simulink model "Simulink_Deliverable"  (R2020a)
settings: Solver=FixedStepAuto  StartTime=0.0  StopTime=10.0  FixedStep=1e-3  RelTol=1e-3  EnableMultiTasking=on
undefined symbols (not defined in the file or in its folder): D0, D1, D10, D11, D12, D13, D2, D3, D4, D5, D6, D7, D8, D9, PTA0, PTA1, PTA2, PTB23, PTB9, PTC16, PTC17, PTC2, PTC3, PTC4, PTD0, PTD1, PTD2, PTD3
libraries: frdmk64flib x17
settings Model: ExtModeTrigDuration=5  Creator=shivr  LastModifiedBy=shivr
settings OptimizationCC: EnhancedBackFolding=on  PassReuseOutputArgsAs=Individual arguments  ZeroExternalMemoryAtStartup=off  ZeroInternalMemoryAtStartup=off  MaxStackSize=64  OptimizeBlockOrder=speed  DifferentSizesBufferReuse=on  OptimizationCustomize=off  EfficientTunableParamExpr=on
settings DebuggingCC: ParameterTunabilityLossMsg=error
settings HardwareCC: ProdBitPerPointer=32  ProdBitPerSizeT=32  ProdBitPerPtrDiffT=32  ProdLargestAtomicInteger=Long  ProdLargestAtomicFloat=Double  ProdWordSize=32  ProdHWDeviceType=ARM Compatible->ARM Cortex
settings SFSimCC: MATLABDynamicMemAlloc=off
settings RTWCC: SystemTargetFile=ert.tlc  HardwareBoard=NXP FRDM-K64F  TemplateMakefile=ert_default_tmf  Toolchain=GNU Tools for ARM Embedded Processors
settings CodeAppCC: ForceParamTrailComments=on  IgnoreCustomStorageClasses=off  OperatorAnnotations=on  SimulinkDataObjDesc=on  SFDataObjDesc=on  InsertBlockDesc=on

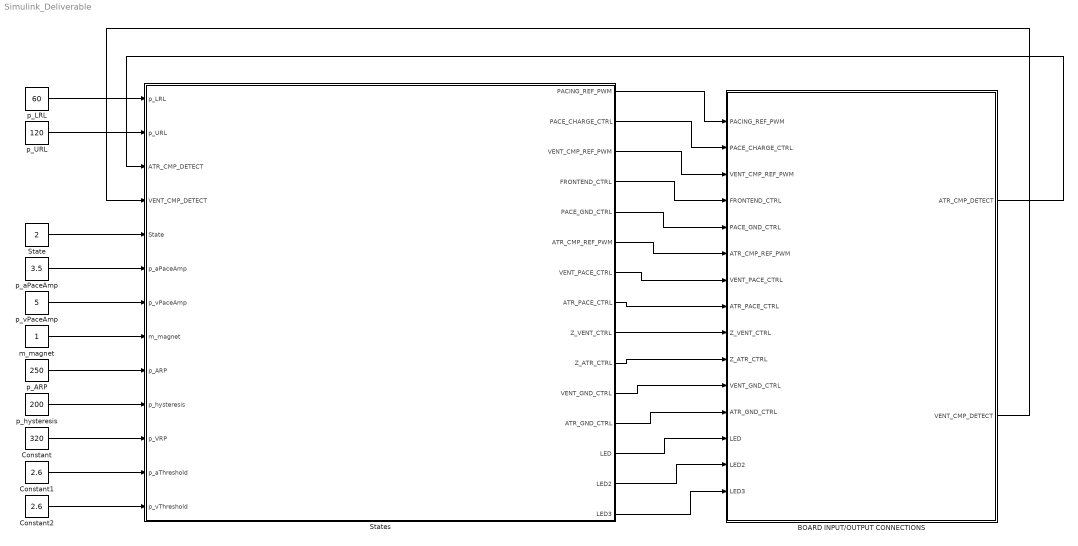
== system Simulink_Deliverable ==
  BOARD INPUT/OUTPUT CONNECTIONS : Subsystem
  Constant : Constant  Value=320
  Constant1 : Constant  Value=2.6
  Constant2 : Constant  Value=2.6
  State : Constant  Value=2
  States : Subsystem
  m_magnet : Constant
  p_ARP : Constant  Value=250
  p_LRL : Constant  Value=60
  p_URL : Constant  Value=120
  p_aPaceAmp : Constant  Value=3.5
  p_hysteresis : Constant  Value=200
  p_vPaceAmp : Constant  Value=5
  wires:
  p_LRL/1 -> States/1(p_LRL)
  States/12(ATR_GND_CTRL) -> BOARD INPUT/OUTPUT CONNECTIONS/12(ATR_GND_CTRL)
  States/5(PACE_GND_CTRL) -> BOARD INPUT/OUTPUT CONNECTIONS/5(PACE_GND_CTRL)
  States/11(VENT_GND_CTRL) -> BOARD INPUT/OUTPUT CONNECTIONS/11(VENT_GND_CTRL)
  States/7(VENT_PACE_CTRL) -> BOARD INPUT/OUTPUT CONNECTIONS/7(VENT_PACE_CTRL)
  States/8(ATR_PACE_CTRL) -> BOARD INPUT/OUTPUT CONNECTIONS/8(ATR_PACE_CTRL)
  States/9(Z_VENT_CTRL) -> BOARD INPUT/OUTPUT CONNECTIONS/9(Z_VENT_CTRL)
  States/10(Z_ATR_CTRL) -> BOARD INPUT/OUTPUT CONNECTIONS/10(Z_ATR_CTRL)
  States/4(FRONTEND_CTRL) -> BOARD INPUT/OUTPUT CONNECTIONS/4(FRONTEND_CTRL)
  States/2(PACE_CHARGE_CTRL) -> BOARD INPUT/OUTPUT CONNECTIONS/2(PACE_CHARGE_CTRL)
  States/1(PACING_REF_PWM) -> BOARD INPUT/OUTPUT CONNECTIONS/1(PACING_REF_PWM)
  States/13(LED) -> BOARD INPUT/OUTPUT CONNECTIONS/13(LED)
  p_URL/1 -> States/2(p_URL)
  BOARD INPUT/OUTPUT CONNECTIONS/1(ATR_CMP_DETECT) -> States/3(ATR_CMP_DETECT)
  BOARD INPUT/OUTPUT CONNECTIONS/2(VENT_CMP_DETECT) -> States/4(VENT_CMP_DETECT)
  p_aPaceAmp/1 -> States/6(p_aPaceAmp)
  m_magnet/1 -> States/8(m_magnet)
  States/14(LED2) -> BOARD INPUT/OUTPUT CONNECTIONS/14(LED2)
  p_vPaceAmp/1 -> States/7(p_vPaceAmp)
  States/6(ATR_CMP_REF_PWM) -> BOARD INPUT/OUTPUT CONNECTIONS/6(ATR_CMP_REF_PWM)
  p_ARP/1 -> States/9(p_ARP)
  p_hysteresis/1 -> States/10(p_hysteresis)
  States/15(LED3) -> BOARD INPUT/OUTPUT CONNECTIONS/15(LED3)
  States/3(VENT_CMP_REF_PWM) -> BOARD INPUT/OUTPUT CONNECTIONS/3(VENT_CMP_REF_PWM)
  Constant/1 -> States/11(p_VRP)
  Constant1/1 -> States/12(p_aThreshold)
  Constant2/1 -> States/13(p_vThreshold)
  State/1 -> States/5(State)

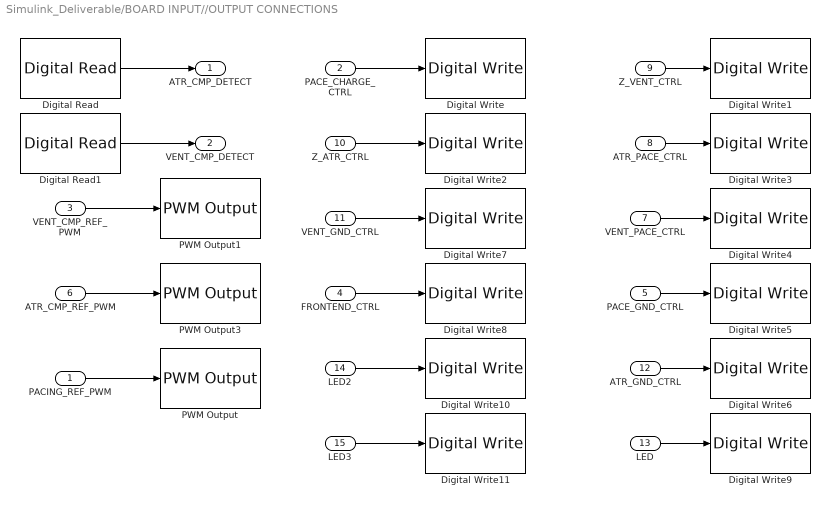
== system Simulink_Deliverable/BOARD INPUT//OUTPUT CONNECTIONS ==
  PACING_REF_PWM : Inport
  PACE_CHARGE_CTRL : Inport  Port=2
  VENT_CMP_REF_PWM : Inport  Port=3
  FRONTEND_CTRL : Inport  Port=4
  PACE_GND_CTRL : Inport  Port=5
  ATR_CMP_REF_PWM : Inport  Port=6
  VENT_PACE_CTRL : Inport  Port=7
  ATR_PACE_CTRL : Inport  Port=8
  Z_VENT_CTRL : Inport  Port=9
  Z_ATR_CTRL : Inport  Port=10
  VENT_GND_CTRL : Inport  Port=11
  ATR_GND_CTRL : Inport  Port=12
  LED : Inport  Port=13
  LED2 : Inport  Port=14
  LED3 : Inport  Port=15
  Digital Read : frdmk64flib/Digital Read  Whichpin=PTC16 (D0)  SampleTime=-1
  Digital Read1 : frdmk64flib/Digital Read  Whichpin=PTC17 (D1)  SampleTime=-1
  Digital Write : frdmk64flib/Digital Write  Whichpin=PTB9 (D2)
  Digital Write1 : frdmk64flib/Digital Write  Whichpin=PTC3 (D7)
  Digital Write10 : frdmk64flib/Digital Write  Whichpin=BLUE_LED
  Digital Write11 : frdmk64flib/Digital Write  Whichpin=GREEN_LED
  Digital Write2 : frdmk64flib/Digital Write  Whichpin=PTB23 (D4)
  Digital Write3 : frdmk64flib/Digital Write  Whichpin=PTA0 (D8)
  Digital Write4 : frdmk64flib/Digital Write  Whichpin=PTC4 (D9)
  Digital Write5 : frdmk64flib/Digital Write  Whichpin=PTD0 (D10)
  Digital Write6 : frdmk64flib/Digital Write  Whichpin=PTD2 (D11)
  Digital Write7 : frdmk64flib/Digital Write  Whichpin=PTD3 (D12)
  Digital Write8 : frdmk64flib/Digital Write  Whichpin=PTD1 (D13)
  Digital Write9 : frdmk64flib/Digital Write  Whichpin=RED_LED
  PWM Output : frdmk64flib/PWM Output  Whichpin=PTA2 (D5)  InitialFrequency=2000  InitialDutyCycle=0
  PWM Output1 : frdmk64flib/PWM Output  Whichpin=PTA1 (D3)  InitialFrequency=2000  InitialDutyCycle=0
  PWM Output3 : frdmk64flib/PWM Output  Whichpin=PTC2 (D6)  InitialFrequency=2000  InitialDutyCycle=100
  ATR_CMP_DETECT : Outport
  VENT_CMP_DETECT : Outport  Port=2
  wires:
  Digital Read/1 -> ATR_CMP_DETECT/1
  Digital Read1/1 -> VENT_CMP_DETECT/1
  VENT_CMP_REF_PWM/1 -> PWM Output1/1
  PACE_CHARGE_CTRL/1 -> Digital Write/1
  Z_ATR_CTRL/1 -> Digital Write2/1
  PACING_REF_PWM/1 -> PWM Output/1
  ATR_CMP_REF_PWM/1 -> PWM Output3/1
  Z_VENT_CTRL/1 -> Digital Write1/1
  ATR_PACE_CTRL/1 -> Digital Write3/1
  VENT_PACE_CTRL/1 -> Digital Write4/1
  PACE_GND_CTRL/1 -> Digital Write5/1
  ATR_GND_CTRL/1 -> Digital Write6/1
  VENT_GND_CTRL/1 -> Digital Write7/1
  FRONTEND_CTRL/1 -> Digital Write8/1
  LED/1 -> Digital Write9/1
  LED2/1 -> Digital Write10/1
  LED3/1 -> Digital Write11/1

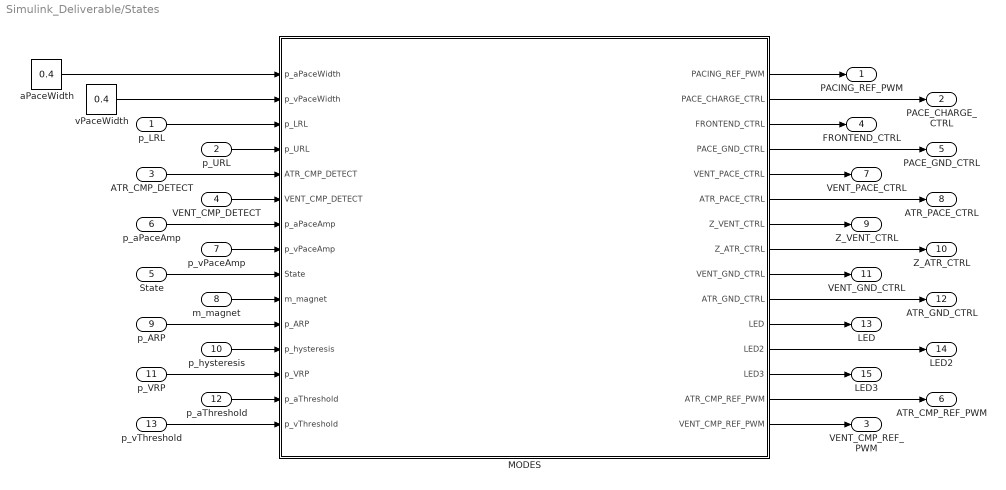
== system Simulink_Deliverable/States ==
  p_LRL : Inport
  p_URL : Inport  Port=2
  ATR_CMP_DETECT : Inport  Port=3
  VENT_CMP_DETECT : Inport  Port=4
  State : Inport  Port=5
  p_aPaceAmp : Inport  Port=6
  p_vPaceAmp : Inport  Port=7
  m_magnet : Inport  Port=8
  p_ARP : Inport  Port=9
  p_hysteresis : Inport  Port=10
  p_VRP : Inport  Port=11
  p_aThreshold : Inport  Port=12
  p_vThreshold : Inport  Port=13
  MODES : Stateflow chart  TreatAsAtomicUnit=on
      settings: PortSchema="{\"entries\":[{\"content\":{\"sides\":[{\"content\":{\"connectorIds\":[\"In1\",\"In2\",\"In3\",\"In4\",\"In5\",\"In6\",\"In7\",\"In8\",\"In9\",\"In10\",\"In11\",\"In12\",\"In13\",\"In14\",\"In15\"]},\"type\":\"ConnectorPlacement.EquallySpacedRectSide\",\"uuid\":\"8502a3c5-6307-4e02-81ee-17e1a35cc298\"},{\"content\":{\"connectorIds\":[\"Out1\",\"Out2\",\"Out3\",\"Out4\",\"Out5\",\"Out6\",\"Out7\",\"Out8\",\"Out9\",\"Out10\",\"Out11\",\"Out14\",\"Out13\",\"Out12\",\"Out15\"],\"side\":\"RIGHT\"},\"type\":\"ConnectorPlacement.EquallySpacedRectSide\",\"uuid\":\"71555ad9-e88e-4949-94fd-af1b739ca2ca\"},{\"content\":{\"connectorIds\":[],\"side\":\"TOP\"},\"type\":\"ConnectorPlacement.EquallySpacedRectSide\",\"uuid\":\"f0239cae-2fc2-4d44-ac00-93735ab3ef8c\"},{\"content\":{\"connectorIds\":[],\"side\":\"BOTTOM\"},\"type\":\"ConnectorPlacement.EquallySpacedRectSide\",\"uuid\":\"7d1612d5-a202-47d8-98e6-e2ca77499232\"}]},\"type\":\"ConnectorPlacement.EquallySpacedConnector\",\"uuid\":\"0a066545-78b2-4ddc-84c3-90461cea3699\"}],\"packageUris\":[\"http://schema.mathworks.com/mf0/Connector/19700101\"],\"version\":\"1.0\"}"
  aPaceWidth : Constant  Value=0.4
  vPaceWidth : Constant  Value=0.4
  PACING_REF_PWM : Outport
  PACE_CHARGE_CTRL : Outport  Port=2
  VENT_CMP_REF_PWM : Outport  Port=3
  FRONTEND_CTRL : Outport  Port=4
  PACE_GND_CTRL : Outport  Port=5
  ATR_CMP_REF_PWM : Outport  Port=6
  VENT_PACE_CTRL : Outport  Port=7
  ATR_PACE_CTRL : Outport  Port=8
  Z_VENT_CTRL : Outport  Port=9
  Z_ATR_CTRL : Outport  Port=10
  VENT_GND_CTRL : Outport  Port=11
  ATR_GND_CTRL : Outport  Port=12
  LED : Outport  Port=13
  LED2 : Outport  Port=14
  LED3 : Outport  Port=15
  wires:
  aPaceWidth/1 -> MODES/1(p_aPaceWidth)
  MODES/5(VENT_PACE_CTRL) -> VENT_PACE_CTRL/1
  MODES/3(FRONTEND_CTRL) -> FRONTEND_CTRL/1
  MODES/1(PACING_REF_PWM) -> PACING_REF_PWM/1
  MODES/6(ATR_PACE_CTRL) -> ATR_PACE_CTRL/1
  MODES/7(Z_VENT_CTRL) -> Z_VENT_CTRL/1
  MODES/4(PACE_GND_CTRL) -> PACE_GND_CTRL/1
  MODES/8(Z_ATR_CTRL) -> Z_ATR_CTRL/1
  MODES/2(PACE_CHARGE_CTRL) -> PACE_CHARGE_CTRL/1
  MODES/9(VENT_GND_CTRL) -> VENT_GND_CTRL/1
  MODES/10(ATR_GND_CTRL) -> ATR_GND_CTRL/1
  MODES/11(LED) -> LED/1
  p_LRL/1 -> MODES/3(p_LRL)
  p_URL/1 -> MODES/4(p_URL)
  ATR_CMP_DETECT/1 -> MODES/5(ATR_CMP_DETECT)
  VENT_CMP_DETECT/1 -> MODES/6(VENT_CMP_DETECT)
  p_aPaceAmp/1 -> MODES/7(p_aPaceAmp)
  m_magnet/1 -> MODES/10(m_magnet)
  MODES/14(LED2) -> LED2/1
  vPaceWidth/1 -> MODES/2(p_vPaceWidth)
  p_vPaceAmp/1 -> MODES/8(p_vPaceAmp)
  MODES/12(ATR_CMP_REF_PWM) -> ATR_CMP_REF_PWM/1
  p_ARP/1 -> MODES/11(p_ARP)
  p_hysteresis/1 -> MODES/12(p_hysteresis)
  MODES/13(LED3) -> LED3/1
  p_VRP/1 -> MODES/13(p_VRP)
  MODES/15(VENT_CMP_REF_PWM) -> VENT_CMP_REF_PWM/1
  p_aThreshold/1 -> MODES/14(p_aThreshold)
  p_vThreshold/1 -> MODES/15(p_vThreshold)
  State/1 -> MODES/9(State)

== stateflow chart Simulink_Deliverable/States/MODES ==
  state AOO
    state Prep
      entry:
      FRONTEND_CTRL=false; %sensing off
      %start charging C22
      ATR_PACE_CTRL = false;       %1
      VENT_PACE_CTRL = false;      %2
      PACING_REF_PWM = p_aPaceAmp/5*100; %3
      PACE_CHARGE_CTRL = true;  %4
      %discharge blocking (combined state)
      PACE_GND_CTRL = true; %
      Z_ATR_CTRL= false;
      Z_VENT_CTRL=false;
      ATR_GND_CTRL = true;
      VENT_GND_CTRL = false;
      LED = false;
    state Pace
      entry:
      PACE_CHARGE_CTRL = false;
      ATR_PACE_CTRL = true;
      ATR_GND_CTRL = false;
      LED = true;
    (default) -> Prep
    Prep -> Pace : [after(60000/p_LRL-p_aPaceWidth, msec)]
    Pace -> Prep : [after(p_aPaceWidth, msec)]
  state VOO
    state VOO_Pace_State
      entry:
      PACE_CHARGE_CTRL=false;
      VENT_GND_CTRL=false;
      VENT_PACE_CTRL=true;
      LED2 = true;
    state VOO_Prep_State
      entry:
      FRONTEND_CTRL=false;
      %charging
      ATR_PACE_CTRL = false;
      VENT_PACE_CTRL=false;
      PACING_REF_PWM = p_vPaceAmp/5*100;
      PACE_CHARGE_CTRL=true;
      %discharging
      PACE_GND_CTRL=true; %vp = 0
      Z_ATR_CTRL = false;
      Z_VENT_CTRL=false;
      ATR_GND_CTRL = false;
      VENT_GND_CTRL=true; %c_vp=0;
      LED2 = false;
    (default) -> VOO_Prep_State
    VOO_Prep_State -> VOO_Pace_State : [after(60000.0/p_LRL - p_vPaceWidth,msec)]
    VOO_Pace_State -> VOO_Prep_State : [after(p_vPaceWidth,msec)]
  state state_selector
  state AAI
    state AAI_CHARGING_DISCHARGING
      entry:
      FRONTEND_CTRL = true; %enable sensing
      %charge
      ATR_PACE_CTRL = false;
      PACE_CHARGE_CTRL = true;
      PACE_GND_CTRL = true;
      VENT_PACE_CTRL = false;
      PACING_REF_PWM = p_aPaceAmp/5*100;
      %discharge
      ATR_GND_CTRL = true;
      VENT_PACE_CTRL = false;
      VENT_GND_CTRL = false;
      Z_ATR_CTRL = false;
      Z_VENT_CTRL = false;
      LED3 = false;
      %Double Check
      ATR_CMP_REF_PWM = p_aThreshold/5*100;
      %52
    state AAI_PACING
      entry:
      %turn off sensing
      FRONTEND_CTRL = false;
      %pace like aoo
      PACE_CHARGE_CTRL = false;
      ATR_PACE_CTRL = true;
      ATR_GND_CTRL = false;
      LED3 = true;
    state AAI_REFRACTORY
      entry:
      LED2 = ~LED2;
    (default) -> AAI_CHARGING_DISCHARGING
    AAI_CHARGING_DISCHARGING -> AAI_PACING [order 1] : [ATR_CMP_DETECT==false&&after((60000/p_LRL-p_aPaceWidth), msec)]
    AAI_PACING -> AAI_CHARGING_DISCHARGING : [after(p_aPaceWidth, msec)]
    AAI_REFRACTORY -> AAI_CHARGING_DISCHARGING : [after(p_ARP, msec)]
    AAI_CHARGING_DISCHARGING -> AAI_REFRACTORY [order 2] : [ATR_CMP_DETECT == true]
  state VVI
    state VVI_SENSING
      entry:
      FRONTEND_CTRL = true; %enable sensing
      %charge
      ATR_PACE_CTRL = false;
      PACE_CHARGE_CTRL = true;
      PACE_GND_CTRL = true;
      VENT_PACE_CTRL = false;
      PACING_REF_PWM = p_vPaceAmp/5*100;
      %discharge
      ATR_GND_CTRL =false;
      VENT_GND_CTRL = true;
      Z_ATR_CTRL = false;
      Z_VENT_CTRL = false;
      LED3 = false;
      %Double Check
      VENT_CMP_REF_PWM = p_vThreshold/5*100;
      %52
    state VVI_PACING
      entry:
      %turn off sensing
      FRONTEND_CTRL = false;
      %pace like VOO
      PACE_CHARGE_CTRL = false;
      PACE_GND_CTRL = true;
      VENT_PACE_CTRL = true;
      VENT_GND_CTRL = false;
      LED3 = true;
    state VVI_REFRACTORY
      entry:
      LED2 = ~LED2;
    (default) -> VVI_SENSING
    VVI_SENSING -> VVI_PACING [order 1] : [VENT_CMP_DETECT==false&&after((60000/p_LRL-p_vPaceWidth), msec)]
    VVI_PACING -> VVI_SENSING : [after(p_vPaceWidth, msec)]
    VVI_REFRACTORY -> VVI_SENSING : [after(p_VRP, msec)]
    VVI_SENSING -> VVI_REFRACTORY [order 2] : [VENT_CMP_DETECT == true]
  state_selector -> AOO [order 1] : [State == 1&&m_magnet==0]
  state_selector -> VOO [order 2] : [m_magnet == 1 || State == 2]
  (default) -> state_selector
  state_selector -> AAI [order 3] : [State == 3&&m_magnet==0]
  state_selector -> VVI [order 4] : [State == 4&&m_magnet==0]
  data: PACING_REF_PWM output; PACE_CHARGE_CTRL output; FRONTEND_CTRL output; PACE_GND_CTRL output; VENT_PACE_CTRL output; ATR_PACE_CTRL output; Z_VENT_CTRL output; Z_ATR_CTRL output; VENT_GND_CTRL output; ATR_GND_CTRL output; LED output; ATR_CMP_REF_PWM output; LED3 output; p_aPaceWidth input; p_vPaceWidth input; p_LRL input; p_URL input; ATR_CMP_DETECT input; VENT_CMP_DETECT input; p_aPaceAmp input; p_vPaceAmp input; State input; m_magnet input; LED2 output; p_ARP input; p_hysteresis input; p_VRP input; VENT_CMP_REF_PWM output; p_aThreshold input; p_vThreshold input
